simulink model "Nonlinear"  (R2019a)
settings: Solver=ode45  StartTime=0.0  StopTime=tf  MaxStep=step  RelTol=tol  AbsTol=tol
values from neighbouring files (symbols this model uses):
  A = [0,                      1,                      0, 0;       0, -(Ip+mp*L^2)*f/s_denom,     g*mp^2*L^2/s_denom, 0;       0,                      0,                      0, 1;       0,        -mp*L*f/s_denom, mp*g*L*(mc+mp)/s_denom, 0]    [SimNonlinear.m]    (also in offset_dynamics.m = simplify(A))
  B = [0; (Ip+mp*L^2)/s_denom; 0; mp*L/s_denom]    [SimNonlinear.m]    (also in offset_dynamics.m = simplify(B))
  C = eye(4)    [SimNonlinear.m]    (also in normal_dynamics.m = simplify(C); offset_dynamics.m)
  D = zeros(4, 1)    [SimNonlinear.m]    (also in offset_dynamics.m)
  dtheta0 = 0    [SimNonlinear.m]
  dx0 = 0    [SimNonlinear.m]
  f = 0.01    [SimNonlinear.m]    (also in animate_2D.m = figure(); normal_dynamics_params.m; normaldyn_fun.m = in3(:,7); offset_dynamics_params.m)
  g = 9.81    [SimNonlinear.m]    (also in normaldyn_fun.m = in3(:,6); offsetdyn_fun.m = in3(:,10))
  init_state = [x0; dx0; theta0; dtheta0]    [SimNonlinear.m]
  Ip = 0.00024    [SimNonlinear.m]    (also in normal_dynamics_params.m; normaldyn_fun.m = in3(:,4); offset_dynamics_params.m; offset_dynamics_sim.m)
  K = lqr(A, B, Q, R)    [SimNonlinear.m]    (also in normal_dyn_controller.mat = [-31.6227766017 -46.3910592069 186.459754798 34.6298374135]; offset_dyn_controller.mat = [-31.6227766017 -46.4351184767 187.329434162 34.9118542309]; offset_dynamics.m = lqr(A_sys, B_sys, Q, R))
  L = 0.04    [SimNonlinear.m]
  mc = 0.493    [SimNonlinear.m]    (also in normal_dynamics_params.m; normaldyn_fun.m = in3(:,3); offset_dynamics_params.m; offset_dynamics_sim.m)
  mp = 0.312    [SimNonlinear.m]    (also in normal_dynamics_params.m; normaldyn_fun.m = in3(:,2); offset_dynamics_params.m; offset_dynamics_sim.m)
  ref = [xr; dxr; thetar; dthetar]    [SimNonlinear.m]
  theta0 = -pi/6    (= -0.523598775598)    [SimNonlinear.m]
  x0 = 1    [SimNonlinear.m]    (also in normal_dynamics_sim.m = [0; 0; -pi/4; 0]; offset_dynamics_sim.m = [0; 0; pi; 0])
settings Model: Creator=bednarse  LastModifiedBy=bednarse
settings DataIOCC: ReturnWorkspaceOutputsName=sdata

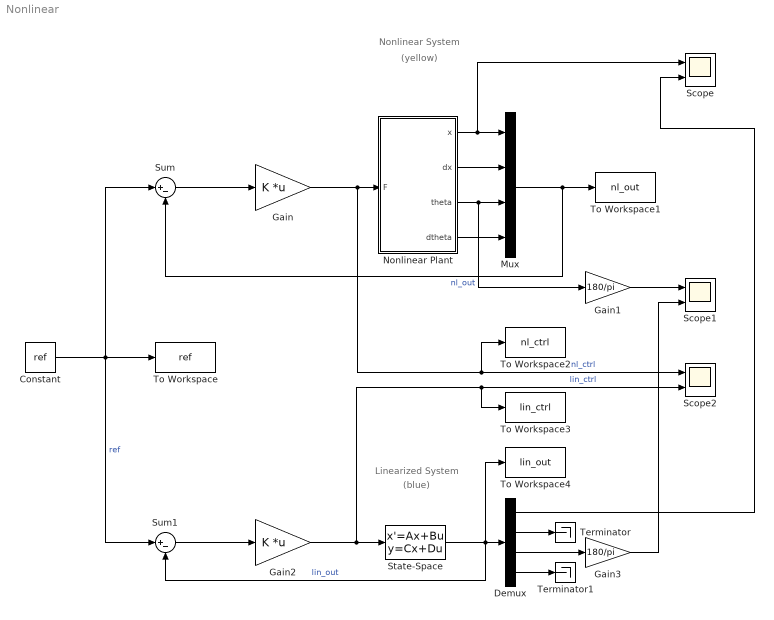
== system Nonlinear ==
  note: Nonlinear System
  note: Linearized System
  note: (yellow)
  note: (blue)
  Constant : Constant  Value=ref
  Demux : Demux
  Gain : Gain  Gain=K  Multiplication=Matrix(K*u) (u vector)
  Gain1 : Gain  Gain=180/pi
  Gain2 : Gain  Gain=K  Multiplication=Matrix(K*u) (u vector)
  Gain3 : Gain  Gain=180/pi
  Mux : Mux
  Nonlinear Plant : Subsystem
  Scope : Scope  NumInputPorts=2
  Scope1 : Scope  NumInputPorts=2
  Scope2 : Scope  NumInputPorts=2
  State-Space : StateSpace  A=A  B=B  C=C  D=D  InitialCondition=init_state
  Sum : Sum  Inputs=|+-
  Sum1 : Sum  Inputs=|+-
  Terminator : Terminator
  Terminator1 : Terminator
  To Workspace : ToWorkspace  VariableName=ref  SampleTime=-1
  To Workspace1 : ToWorkspace  VariableName=nl_out  SampleTime=-1
  To Workspace2 : ToWorkspace  VariableName=nl_ctrl  SampleTime=-1
  To Workspace3 : ToWorkspace  VariableName=lin_ctrl  SampleTime=-1
  To Workspace4 : ToWorkspace  VariableName=lin_out  SampleTime=-1
  wires:
  Gain/1 -> To Workspace2/1, Scope2/1, Nonlinear Plant/1(F)  "nl_ctrl"
  Nonlinear Plant/1(x) -> Scope/1, Mux/1
  Nonlinear Plant/2(dx) -> Mux/2
  Nonlinear Plant/3(theta) -> Gain1/1, Mux/3
  Nonlinear Plant/4(dtheta) -> Mux/4
  Gain1/1 -> Scope1/1
  Gain2/1 -> To Workspace3/1, Scope2/2, State-Space/1  "lin_ctrl"
  State-Space/1 -> To Workspace4/1, Demux/1, Sum1/2  "lin_out"
  Demux/2 -> Terminator/1
  Demux/4 -> Terminator1/1
  Demux/3 -> Gain3/1
  Gain3/1 -> Scope1/2
  Sum1/1 -> Gain2/1
  Mux/1 -> To Workspace1/1, Sum/2  "nl_out"
  Sum/1 -> Gain/1
  Constant/1 -> To Workspace/1, Sum1/1, Sum/1  "ref"
  Demux/1 -> Scope/2

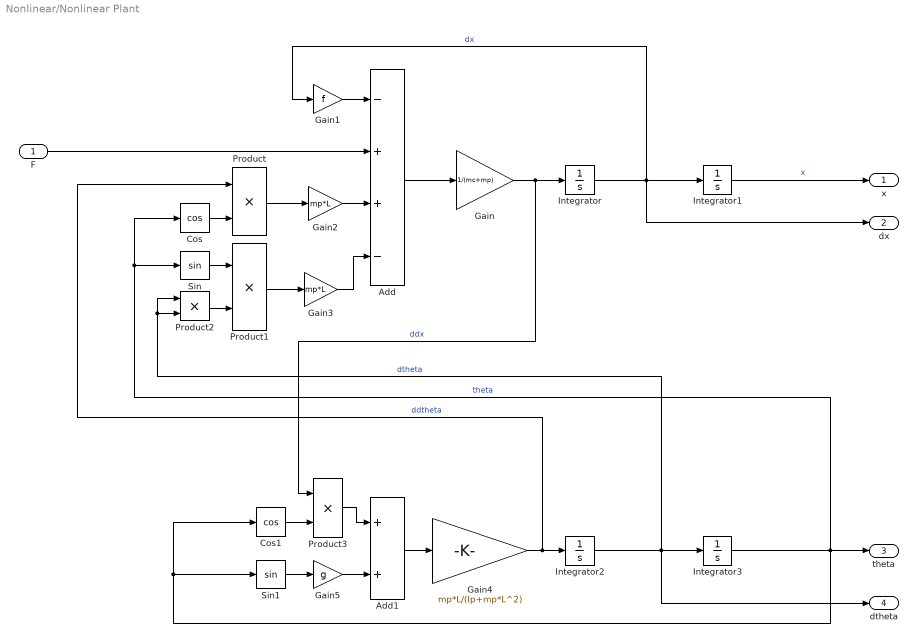
== system Nonlinear/Nonlinear Plant ==
  F : Inport
  Add : Sum  Inputs=-++-
  Add1 : Sum
  Cos : Trigonometry  Operator=cos
  Cos1 : Trigonometry  Operator=cos
  Gain : Gain  Gain=1/(mc+mp)
  Gain1 : Gain  Gain=f
  Gain2 : Gain  Gain=mp*L
  Gain3 : Gain  Gain=mp*L
  Gain4 : Gain  Gain=mp*L/(Ip+mp*L^2)
  Gain5 : Gain  Gain=g
  Integrator : Integrator  InitialCondition=dx0
  Integrator1 : Integrator  InitialCondition=x0
  Integrator2 : Integrator  InitialCondition=dtheta0
  Integrator3 : Integrator  InitialCondition=theta0
  Product{,1..3} (4 alike) : Product
  Sin : Trigonometry
  Sin1 : Trigonometry
  x : Outport
  dx : Outport  Port=2
  theta : Outport  Port=3
  dtheta : Outport  Port=4
  wires:
  Integrator/1 -> Integrator1/1, dx/1, Gain1/1  "dx"
  Integrator2/1 -> Product2/1, Product2/2, dtheta/1, Integrator3/1  "dtheta"
  Gain/1 -> Product3/1, Integrator/1  "ddx"
  Add/1 -> Gain/1
  Gain1/1 -> Add/1
  F/1 -> Add/2
  Product/1 -> Gain2/1
  Gain3/1 -> Add/4
  Gain2/1 -> Add/3
  Gain4/1 -> Product/1, Integrator2/1  "ddtheta"
  Cos/1 -> Product/2
  Product1/1 -> Gain3/1
  Sin/1 -> Product1/1
  Product2/1 -> Product1/2
  Add1/1 -> Gain4/1
  Sin1/1 -> Gain5/1
  Gain5/1 -> Add1/2
  Product3/1 -> Add1/1
  Cos1/1 -> Product3/2
  Integrator1/1 -> x/1  "x"
  Integrator3/1 -> Cos/1, Sin/1, Cos1/1, Sin1/1, theta/1  "theta"
